simulink model "NestedChartBlock"  (Simulink 7.4)
settings: Solver=ode45  StartTime=0.0  StopTime=10.0  RelTol=1e-3
settings Model: Creator=dread  LastModifiedBy=dread

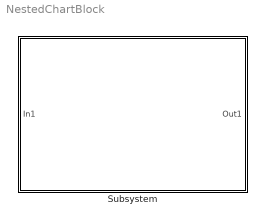
== system NestedChartBlock ==
  Subsystem : Subsystem

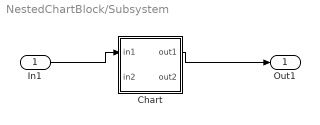
== system NestedChartBlock/Subsystem ==
  In1 : Inport  OutDataType=fixdt(1, 16)  OutScaling=2^0
  Chart : Stateflow chart
  Out1 : Outport  OutDataType=fixdt(1, 16)  OutScaling=2^0
  wires:
  In1/1 -> Chart/1(in1)
  Chart/1(out1) -> Out1/1

== stateflow chart Subsystem/Chart ==
  data: in1 input double; out1 output double; in2 input double; out2 output double
